simulink model "adrc_han"  (R2021a)
settings: Solver=FixedStepDiscrete  StartTime=0.0  StopTime=10.0  FixedStep=0.001  RelTol=1e-3
undefined symbols (not defined in the file or in its folder): DiscIntNeverNeededParam
settings Model: Creator=onqi  LastModifiedBy=root

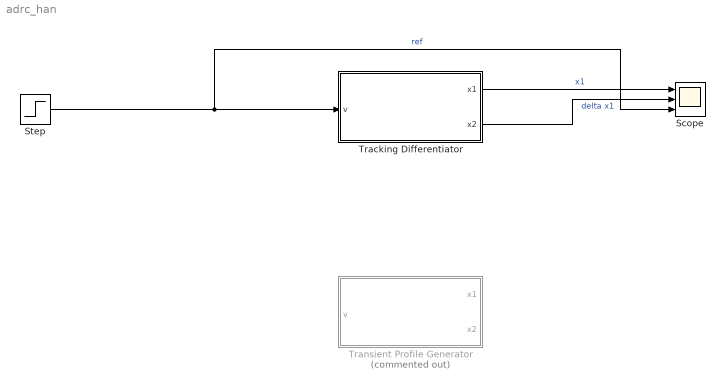
== system adrc_han ==
  Scope : Scope  NumInputPorts=3
  Step : Step  Time=3  SampleTime=0.001
  Tracking Differentiator : Subsystem  SystemSampleTime=SystemSampleTime  mask{r0=10, h0=100, SystemSampleTime=-1}
      mask prompts: r0 "Tracking speed r0"; h0 "Tracking smoothness h0"; SystemSampleTime "Simulink:blkprm_prompts:AllBlksSampleTime"
      mask init:
      | h = str2num(get_param(gcs,'FixedStep'));
      mask TypeOptions SystemSampleTime: SystemSampleTime
      mask DialogControl SystemSampleTime Prompt: Sample time (-1 for inherited):
      mask Display:
      | disp('Tracking Differentiator')
      | port_label('input', 1, '\vee', 'texmode', 'on');
      | port_label('output', 1, 'x_1', 'texmode', 'on');
      | port_label('output', 2, '\Deltax_1', 'texmode', 'on');
  Transient Profile Generator : Subsystem  Commented=on  SystemSampleTime=SystemSampleTime  mask{r=10, SystemSampleTime=-1}
      mask prompts: r "Upper-bound r"; SystemSampleTime "Simulink:blkprm_prompts:AllBlksSampleTime"
      mask init:
      | h = str2num(get_param(gcs,'FixedStep'));
      mask TypeOptions SystemSampleTime: SystemSampleTime
      mask DialogControl SystemSampleTime Prompt: Sample time (-1 for inherited):
      mask Display:
      | disp('Tracking Differentiator')
      | port_label('input', 1, '\vee', 'texmode', 'on');
      | port_label('output', 1, 'x_1', 'texmode', 'on');
      | port_label('output', 2, '\Deltax_1', 'texmode', 'on');
  wires:
  Tracking Differentiator/1(x1) -> Scope/1  "x1"
  Tracking Differentiator/2(x2) -> Scope/2  "delta x1"
  Step/1 -> Scope/3, Tracking Differentiator/1(v)  "ref"

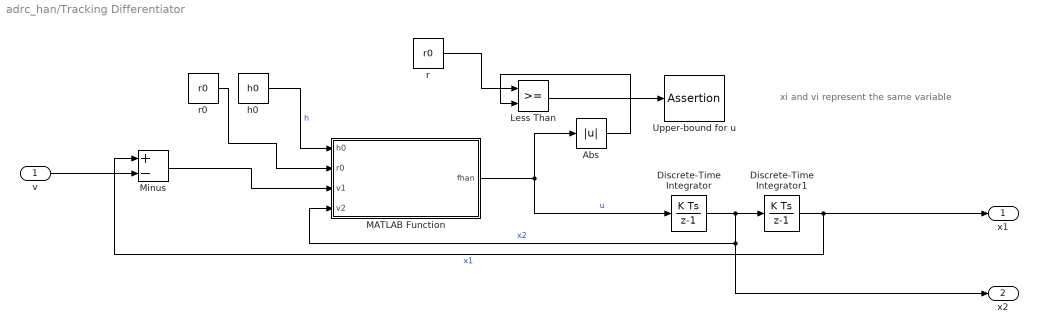
== system adrc_han/Tracking Differentiator ==
  note: xi and vi represent the same variable
  v : Inport
  Abs : Abs
  Discrete-Time Integrator : DiscreteIntegrator  SampleTime=-1  ICPrevOutput=DiscIntNeverNeededParam  ICPrevScaledInput=DiscIntNeverNeededParam
  Discrete-Time Integrator1 : DiscreteIntegrator  SampleTime=-1  ICPrevOutput=DiscIntNeverNeededParam  ICPrevScaledInput=DiscIntNeverNeededParam
  Less Than : RelationalOperator  OutDataTypeStr=boolean  RndMeth=Simplest
  MATLAB Function : MATLAB Function  TreatAsAtomicUnit=on
  Minus : Sum  Inputs=+-
  Upper-bound for u : Assertion
  h0 : Constant  Value=h0  SampleTime=-1
  r : Constant  Value=r0  SampleTime=-1
  r0 : Constant  Value=r0  SampleTime=-1
  x1 : Outport
  x2 : Outport  Port=2
  wires:
  Abs/1 -> Less Than/2
  Less Than/1 -> Upper-bound for u/1
  Discrete-Time Integrator1/1 -> x1/1, Minus/1  "x1"
  Discrete-Time Integrator/1 -> x2/1, MATLAB Function/4(v2), Discrete-Time Integrator1/1  "x2"
  MATLAB Function/1(fhan) -> Discrete-Time Integrator/1, Abs/1  "u"
  Minus/1 -> MATLAB Function/3(v1)
  v/1 -> Minus/2
  r/1 -> Less Than/1
  r0/1 -> MATLAB Function/2(r0)
  h0/1 -> MATLAB Function/1(h0)  "h"

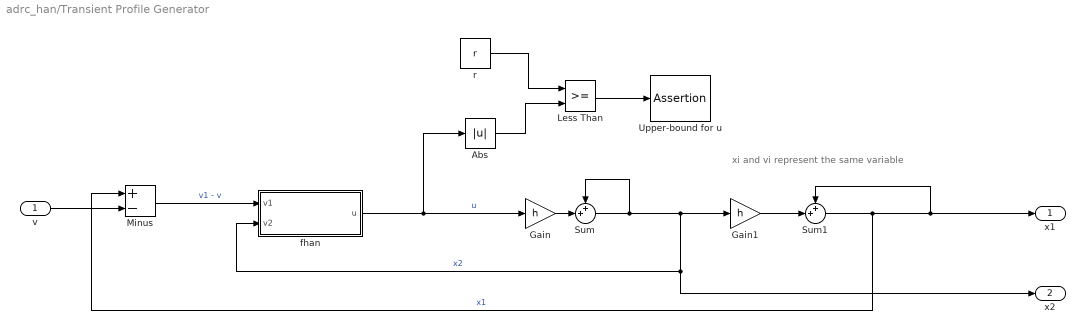
== system adrc_han/Transient Profile Generator ==
  note: xi and vi represent the same variable
  v : Inport
  Abs : Abs
  Gain : Gain  Gain=h
  Gain1 : Gain  Gain=h
  Less Than : RelationalOperator  OutDataTypeStr=boolean  RndMeth=Simplest
  Minus : Sum  Inputs=+-
  Sum : Sum  Inputs=++|
  Sum1 : Sum  Inputs=++|
  Upper-bound for u : Assertion
  fhan : Subsystem
  r : Constant  Value=r  SampleTime=-1
  x1 : Outport
  x2 : Outport  Port=2
  wires:
  Abs/1 -> Less Than/2
  Less Than/1 -> Upper-bound for u/1
  Sum1/1 -> x1/1, Sum1/1, Minus/1  "x1"
  Sum/1 -> x2/1, fhan/2(v2), Gain1/1, Sum/1  "x2"
  fhan/1(u) -> Gain/1, Abs/1  "u"
  Minus/1 -> fhan/1(v1)  "v1 - v"
  v/1 -> Minus/2
  r/1 -> Less Than/1
  Gain/1 -> Sum/2
  Gain1/1 -> Sum1/2

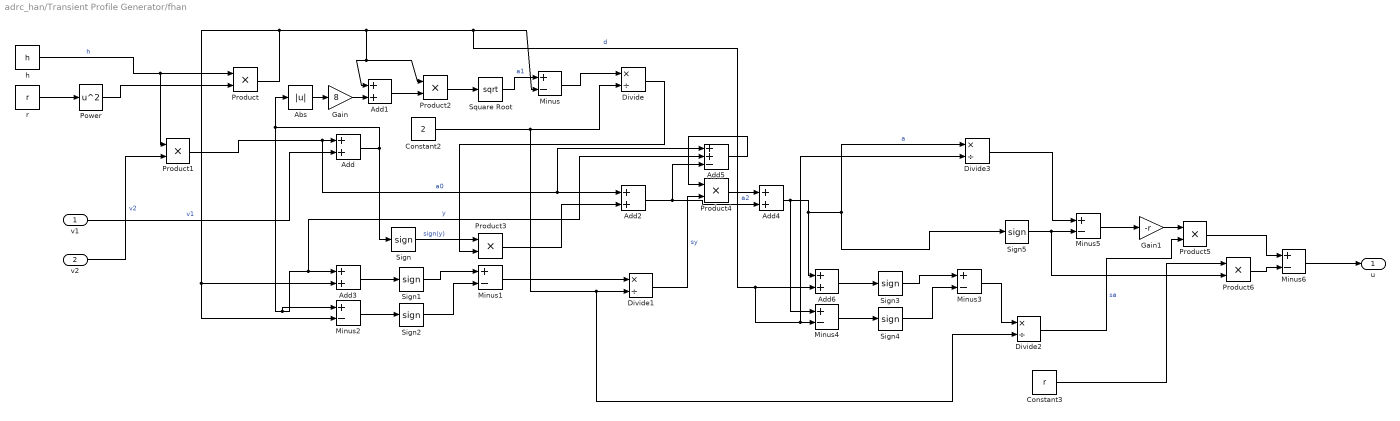
== system adrc_han/Transient Profile Generator/fhan ==
  v1 : Inport
  v2 : Inport  Port=2
  Abs : Abs
  Add{,1..4,6} (6 alike) : Sum
  Add5 : Sum  Inputs=++-
  Constant2 : Constant  Value=2  SampleTime=-1
  Constant3 : Constant  Value=r  SampleTime=-1
  Divide{,1..3} (4 alike) : Product  Inputs=*/
  Gain : Gain  Gain=8
  Gain1 : Gain  Gain=-r
  Minus{,1..6} (7 alike) : Sum  Inputs=+-
  Power : Math  Operator=square  SaturateOnIntegerOverflow=on
  Product{,1..6} (7 alike) : Product
  Sign{,1..5} (6 alike) : Signum
  Square Root : Sqrt  SaturateOnIntegerOverflow=on
  h : Constant  Value=h  SampleTime=-1
  r : Constant  Value=r  SampleTime=-1
  u : Outport
  wires:
  r/1 -> Power/1
  Power/1 -> Product/2
  h/1 -> Product1/1, Product/1  "h"
  Product/1 -> Divide3/2, Minus4/2, Add6/2, Minus/2, Product2/1, Add1/1, Minus2/2, Add3/2  "d"
  v2/1 -> Product1/2  "v2"
  Product1/1 -> Add5/1, Add2/1, Add/1  "a0"
  v1/1 -> Add/2  "v1"
  Add/1 -> Sign/1, Abs/1, Minus2/1, Add5/2, Add3/1  "y"
  Abs/1 -> Gain/1
  Gain/1 -> Add1/2
  Add1/1 -> Product2/2
  Product2/1 -> Square Root/1
  Square Root/1 -> Minus/1  "a1"
  Add2/1 -> Add5/3, Add4/2  "a2"
  Minus/1 -> Divide/1
  Sign/1 -> Product3/1  "sign(y)"
  Divide/1 -> Product3/2
  Product3/1 -> Add2/2
  Sign1/1 -> Minus1/1
  Sign2/1 -> Minus1/2
  Divide1/1 -> Product4/2  "sy"
  Add3/1 -> Sign1/1
  Minus2/1 -> Sign2/1
  Minus1/1 -> Divide1/1
  Add5/1 -> Product4/1
  Product4/1 -> Add4/1
  Add4/1 -> Minus4/1, Sign5/1, Divide3/1, Add6/1  "a"
  Minus4/1 -> Sign4/1
  Add6/1 -> Sign3/1
  Minus3/1 -> Divide2/1
  Sign3/1 -> Minus3/1
  Constant2/1 -> Divide2/2, Divide1/2, Divide/2
  Sign4/1 -> Minus3/2
  Divide2/1 -> Product5/2  "sa"
  Divide3/1 -> Minus5/1
  Sign5/1 -> Product6/2, Minus5/2
  Minus5/1 -> Gain1/1
  Gain1/1 -> Product5/1
  Product5/1 -> Minus6/1
  Constant3/1 -> Product6/1
  Product6/1 -> Minus6/2
  Minus6/1 -> u/1

== matlab function adrc_han/Tracking Differentiator/MATLAB Function ==
  settings: updateMethod=DISCRETE
  data: h0 input; r0 input; v1 input; v2 input; fhan output
function fhan = fhan(h0, r0, v1, v2)

persistent d a0 y a1 a2 sy sa a

if isempty(d)
    d = 0;
end

d = h0*r0^2;
a0 = h0*v2;
y = v1 * a0;

a1 = sqrt(d*(d + 8*abs(y)));
a2 = a0 + sign(y)*(a1 - d)/2;
sy = (sign(y + d) - sign(y - d))/2;
a = (a0 + y - a2)*sy + a2;
sa = (sign(a + d) - sign(a - d))/2;
fhan = -r0*(a/d - sign(a))*sa - r0*sign(a);
